simulink model "ex00_model"  (R2023a)
settings: Solver=FixedStepDiscrete  StartTime=0.0  StopTime=Ts*1e5  RelTol=1e-3
values from neighbouring files (symbols this model uses):
  A0 = 1    [ex00_config.m]
  A1 = 1/4    (= 0.25)    [ex00_config.m]
  Fc0 = +1/8*Fs    (= 125000)    [ex00_config.m]
  Fc1 = -3/8*Fs    (= -375000)    [ex00_config.m]
  hb = buffer(h,2)    [ex00_config.m]
  M = 2    [ex00_config.m]
  Ts = 1/Fs    (= 1e-06)    [ex00_config.m]
libraries: dspsrcs4 x3
settings Model: Creator=daniele  LastModifiedBy=daniele

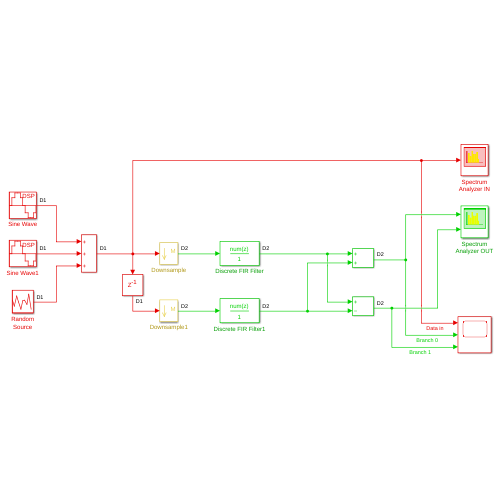
[thumbnail: Simulink's stored preview of the top-level diagram]
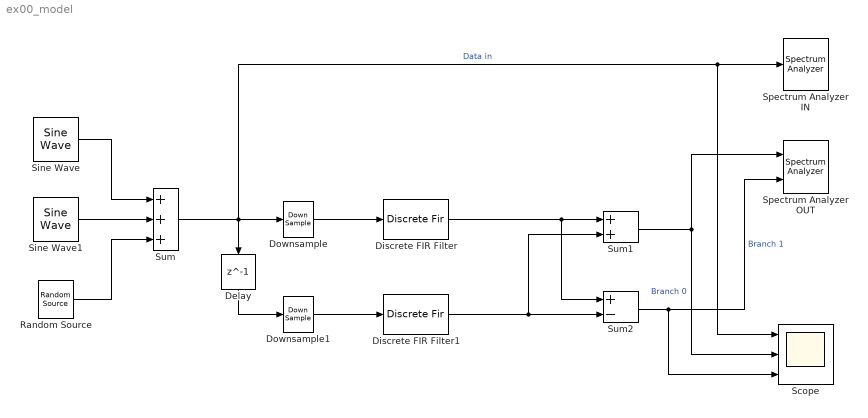
== system ex00_model ==
  Delay : Delay  DelayLength=1
  Discrete FIR Filter : DiscreteFir  Coefficients=hb(1,:)
  Discrete FIR Filter1 : DiscreteFir  Coefficients=hb(2,:)
  Downsample : DownSample  N=M  RateOptions=Allow multirate processing
  Downsample1 : DownSample  N=M  RateOptions=Allow multirate processing
  Random Source : dspsrcs4/Random Source  SrcType=Gaussian  NormMethod=Ziggurat  CltLength=12  MinVal=0  MaxVal=1  MeanVal=0  VarVal=0.01  RepMode=Not repeatable  rawSeed=1  IsInherit=off  SampMode=Discrete  SampTime=Ts  SampFrame=1  DataType=Double  OutComplex=Complex  OutputFrames=off
  Scope : Scope  NumInputPorts=3
  Sine Wave : dspsrcs4/Sine Wave  Amplitude=A0  Frequency=Fc0  Phase=0  SampleMode=Discrete  OutComplex=Complex  CompMethod=Trigonometric fcn  TableSize=Speed  SampleTime=Ts  SamplesPerFrame=1  ResetState=Restart at time zero  OutputFrames=off  dataType=double  wordLen=16  udDataType=sfix(16)  fracBitsMode=Best precision  numFracBits=15  OutDataTypeStr=double  LastOutDataTypeStr=double
  Sine Wave1 : dspsrcs4/Sine Wave  Amplitude=A1  Frequency=Fc1  Phase=0  SampleMode=Discrete  OutComplex=Complex  CompMethod=Trigonometric fcn  TableSize=Speed  SampleTime=Ts  SamplesPerFrame=1  ResetState=Restart at time zero  OutputFrames=off  dataType=double  wordLen=16  udDataType=sfix(16)  fracBitsMode=Best precision  numFracBits=15  OutDataTypeStr=double  LastOutDataTypeStr=double
  Spectrum Analyzer IN : SpectrumAnalyzer  WindowPosition=[101.000000,37.000000,800.000000,500.000000,]  ScopeFrameLocation=window  Span=1000000  StartFrequency=-500000  StopFrequency=500000  YLimits=[-30.72041692,36.74691054]  ColorLimits=[-20 80]  ShowLegend=on  ExpandToolstrip=on  DefaultConfigurationName=spbscopes.SpectrumAnalyzerBlockCfg  IsFrequencyInputMode=0  FrequencyVectorPort=0  FrequencyVectorFromPort=0  FrequencyInputRBWPort=0  FrequencyInputRBWFromPort=0
  Spectrum Analyzer OUT : SpectrumAnalyzer  NumInputPorts=2  WindowPosition=[935.000000,169.000000,800.000000,500.000000,]  ScopeFrameLocation=window  Span=500000  StartFrequency=-250000  StopFrequency=250000  YLimits=[-35.77437624,37.27356447]  ColorLimits=[-20 80]  ShowLegend=on  ExpandToolstrip=on  DefaultConfigurationName=spbscopes.SpectrumAnalyzerBlockCfg  IsFrequencyInputMode=0  FrequencyVectorPort=0  FrequencyVectorFromPort=0  FrequencyInputRBWPort=0  FrequencyInputRBWFromPort=0
  Sum : Sum  Inputs=+++
  Sum1 : Sum
  Sum2 : Sum  Inputs=+-
  wires:
  Sine Wave1/1 -> Sum/2
  Sine Wave/1 -> Sum/1
  Sum/1 -> Spectrum Analyzer IN/1, Scope/1, Delay/1, Downsample/1  "Data in"
  Delay/1 -> Downsample1/1
  Downsample1/1 -> Discrete FIR Filter1/1
  Discrete FIR Filter/1 -> Sum2/1, Sum1/1
  Discrete FIR Filter1/1 -> Sum2/2, Sum1/2
  Downsample/1 -> Discrete FIR Filter/1
  Sum1/1 -> Spectrum Analyzer OUT/1, Scope/2  "Branch 0"
  Sum2/1 -> Scope/3, Spectrum Analyzer OUT/2  "Branch 1"
  Random Source/1 -> Sum/3
